simulink model "NGGenset_Test_System"  (Simulink 8.1)
settings: Solver=ode3  SolverMode=SingleTasking  StartTime=0.0  StopTime=150  FixedStep=Ts  RelTol=1e-3
PostLoadFcn:
  | Ts=50e-6;
InitFcn:
  | Ts=50e-6;
undefined symbols (not defined in the file): another_event_name, DiscIntNeverNeededParam, fdesignblkfcn, gcbh, Gen_900kW_external_control, HIL_GenSet, Left, my_event_name, ph, type, V
libraries: powerlib x47, simulink x40, powerlib_extras x28, rtio_opalrt_common x21, dspsigops x7, breakers_1ph_3ph x7, rtio_generic_modbus x7, simulink_extras x6, cables_lib x5, rteventslib x4, rtlab x3, discretizing x2
(part 3 of 5)

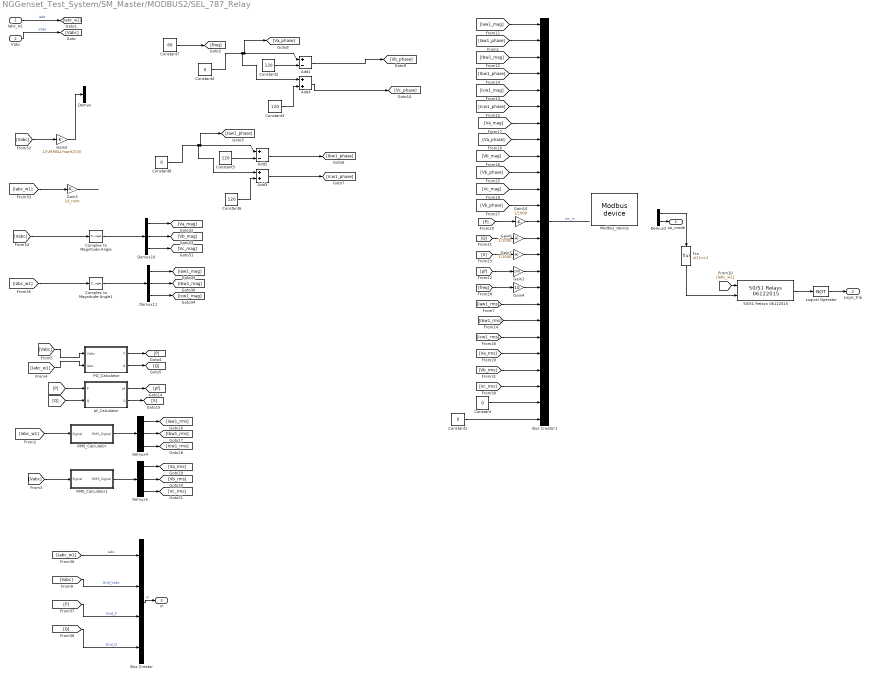
== system NGGenset_Test_System/SM_Master/MODBUS2/SEL_787_Relay ==
  Iabc_w1 : Inport
  Vabc : Inport  Port=2
  50/51 Relays 06122015 : breakers_1ph_3ph/50//51 Relays 06122015  TOC=TOC  IOC=IOC  Ts=Ts
  Add1 : Sum  Inputs=+-
  Add2 : Sum  Inputs=+-
  Add3 : Sum
  Add4 : Sum
  Bus Creator : BusCreator
  Bus Creator1 : BusCreator  Inputs=25
  Complex to Magnitude-Angle : ComplexToMagnitudeAngle  Output=Magnitude
  Complex to Magnitude-Angle1 : ComplexToMagnitudeAngle  Output=Magnitude
  Constant{,1,4,8} (4 alike) : Constant  Value=0
  Constant{2..3,5..6} (4 alike) : Constant  Value=120
  Constant7 : Constant  Value=60
  Demux{,4..5,10..11} (5 alike) : Demux  Outputs=3
  Demux2 : Demux  Outputs=2
  Fcn : Fcn  Expr=u(1)==1
  Gain1 : Gain  Gain=100
  Gain10 : Gain  Gain=1/1000
  Gain2 : Gain  Gain=1/(VRMSLL*sqrt(2/3))
  Gain3 : Gain  Gain=1/I_nom
  Gain4 : Gain  Gain=10
  Gain6 : Gain  Gain=1/1000
  Gain7 : Gain  Gain=1/1000
  Logical Operator : Logic  Operator=NOT  AllPortsSameDT=off  OutDataTypeStr=boolean
  Modbus_device : rtio_generic_modbus/Modbus device  conf_name=relay_slave_cfg2.opal  conf_name_mask=relay_slave_cfg2.xls  sample_time=Ts
  PQ_Calculator : Subsystem
  RMS_Calculator : Subsystem
  RMS_Calculator1 : Subsystem
  pf_Calculator : Subsystem
  op_mode : Outport
  Logic_trip : Outport  Port=2
  m : Outport  Port=3
  wires:
  Gain4/1 -> Bus Creator1/17
  Gain1/1 -> Bus Creator1/16
  [pf] -> Gain1/1
  [freq] -> Gain4/1
  Constant4/1 -> Add4/1, [Va_phase], Add1/1
  Add4/1 -> [Vc_phase]
  Add1/1 -> [Vb_phase]
  Constant3/1 -> Add4/2
  Constant2/1 -> Add1/2
  Constant8/1 -> Add3/1, [Iaw1_phase], Add2/1
  Add3/1 -> [Icw1_phase]
  Add2/1 -> [Ibw1_phase]
  Constant6/1 -> Add3/2
  Constant5/1 -> Add2/2
  Constant7/1 -> [freq]
  pf_Calculator/2(S) -> [S]
  Bus Creator1/1 -> ?  "sm_in"
  ? -> Demux2/1
  [Q] -> Bus Creator/4  "Grid_Q"
  [P] -> Bus Creator/3  "Grid_P"
  [Vabc] -> Bus Creator/2  "Grid_Vabc"
  [Iabc_w1] -> Bus Creator/1  "Iabc"
  Bus Creator/1 -> m/1  "m"
  Iabc_w1/1 -> [Iabc_w1]  "Iabc"
  Vabc/1 -> [Vabc]  "Vabc"
  [Vabc] -> PQ_Calculator/1(Vabc)
  [Iabc_w1] -> PQ_Calculator/2(Iabc)
  [Iaw1_mag] -> Bus Creator1/1
  [P] -> Gain10/1
  [Q] -> Gain6/1
  [S] -> Gain7/1
  pf_Calculator/1(pf) -> [pf]
  [P] -> pf_Calculator/1(P)
  [Q] -> pf_Calculator/2(Q)
  PQ_Calculator/1(P) -> [P]
  PQ_Calculator/2(Q) -> [Q]
  [Iabc_w1] -> RMS_Calculator/1(Signal)
  [Vabc] -> RMS_Calculator1/1(Signal)
  RMS_Calculator/1(RMS_Signal) -> Demux4/1
  RMS_Calculator1/1(RMS_Signal) -> Demux5/1
  Demux4/3 -> [Icw1_rms]
  Demux4/2 -> [Ibw1_rms]
  Demux4/1 -> [Iaw1_rms]
  Demux5/1 -> [Va_rms]
  Demux5/2 -> [Vb_rms]
  Demux5/3 -> [Vc_rms]
  Demux2/1 -> Fcn/1
  Fcn/1 -> 50/51 Relays 06122015/2
  [Iabc_w1] -> 50/51 Relays 06122015/1
  50/51 Relays 06122015/1 -> Logical Operator/1
  [Ibw1_mag] -> Bus Creator1/3
  [Icw1_mag] -> Bus Creator1/5
  [Va_mag] -> Bus Creator1/7
  [Vb_mag] -> Bus Creator1/9
  [Vc_mag] -> Bus Creator1/11
  Gain10/1 -> Bus Creator1/13
  Gain6/1 -> Bus Creator1/14
  Gain7/1 -> Bus Creator1/15
  [Iaw1_rms] -> Bus Creator1/18
  [Icw1_rms] -> Bus Creator1/20
  [Ibw1_rms] -> Bus Creator1/19
  [Va_rms] -> Bus Creator1/21
  [Vb_rms] -> Bus Creator1/22
  [Vc_rms] -> Bus Creator1/23
  Logical Operator/1 -> Logic_trip/1
  Demux2/2 -> op_mode/1
  [Iaw1_phase] -> Bus Creator1/2
  [Ibw1_phase] -> Bus Creator1/4
  [Icw1_phase] -> Bus Creator1/6
  [Va_phase] -> Bus Creator1/8
  [Vb_phase] -> Bus Creator1/10
  [Vb_phase] -> Bus Creator1/12
  Constant/1 -> Bus Creator1/24
  Constant1/1 -> Bus Creator1/25
  [Vabc] -> Gain2/1
  Gain2/1 -> Demux/1
  [Iabc_w1] -> Gain3/1
  Gain3/1 -> ?
  Demux10/1 -> [Va_mag]
  Demux10/2 -> [Vb_mag]
  Demux10/3 -> [Vc_mag]
  Complex to Magnitude-Angle/1 -> Demux10/1
  [Vabc] -> Complex to Magnitude-Angle/1
  Complex to Magnitude-Angle1/1 -> Demux11/1
  [Iabc_w1] -> Complex to Magnitude-Angle1/1
  Demux11/1 -> [Iaw1_mag]
  Demux11/2 -> [Ibw1_mag]
  Demux11/3 -> [Icw1_mag]

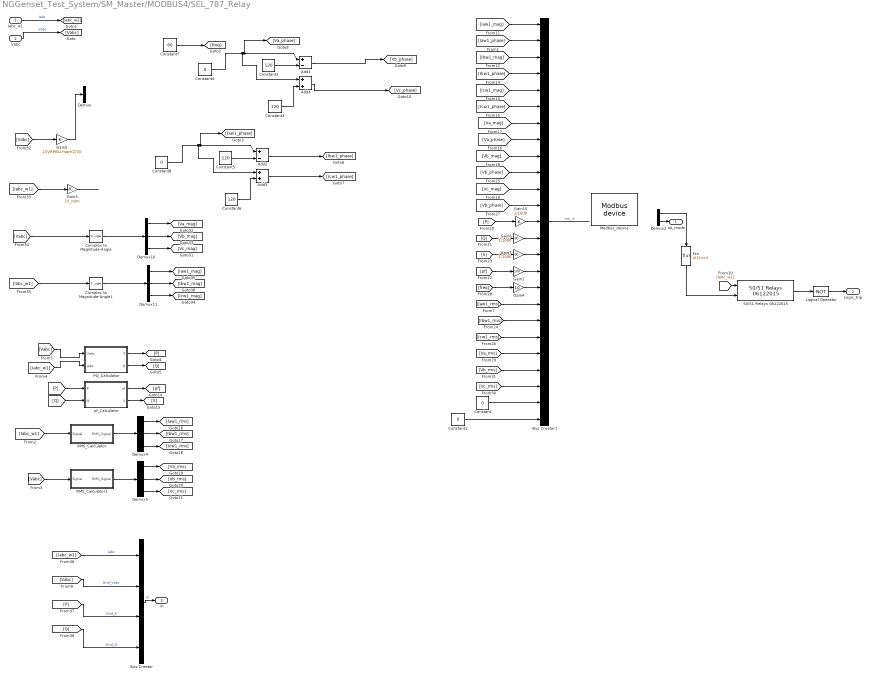
== system NGGenset_Test_System/SM_Master/MODBUS4/SEL_787_Relay ==
  Iabc_w1 : Inport
  Vabc : Inport  Port=2
  50/51 Relays 06122015 : breakers_1ph_3ph/50//51 Relays 06122015  TOC=TOC  IOC=IOC  Ts=Ts
  Add1 : Sum  Inputs=+-
  Add2 : Sum  Inputs=+-
  Add3 : Sum
  Add4 : Sum
  Bus Creator : BusCreator
  Bus Creator1 : BusCreator  Inputs=25
  Complex to Magnitude-Angle : ComplexToMagnitudeAngle  Output=Magnitude
  Complex to Magnitude-Angle1 : ComplexToMagnitudeAngle  Output=Magnitude
  Constant{,1,4,8} (4 alike) : Constant  Value=0
  Constant{2..3,5..6} (4 alike) : Constant  Value=120
  Constant7 : Constant  Value=60
  Demux{,4..5,10..11} (5 alike) : Demux  Outputs=3
  Demux2 : Demux  Outputs=2
  Fcn : Fcn  Expr=u(1)==1
  Gain1 : Gain  Gain=100
  Gain10 : Gain  Gain=1/1000
  Gain2 : Gain  Gain=1/(VRMSLL*sqrt(2/3))
  Gain3 : Gain  Gain=1/I_nom
  Gain4 : Gain  Gain=10
  Gain6 : Gain  Gain=1/1000
  Gain7 : Gain  Gain=1/1000
  Logical Operator : Logic  Operator=NOT  AllPortsSameDT=off  OutDataTypeStr=boolean
  Modbus_device : rtio_generic_modbus/Modbus device  conf_name=relay_slave_cfg4.opal  conf_name_mask=relay_slave_cfg4.xls  sample_time=Ts
  PQ_Calculator : Subsystem
  RMS_Calculator : Subsystem
  RMS_Calculator1 : Subsystem
  pf_Calculator : Subsystem
  op_mode : Outport
  Logic_trip : Outport  Port=2
  m : Outport  Port=3
  wires:
  Gain4/1 -> Bus Creator1/17
  Gain1/1 -> Bus Creator1/16
  [pf] -> Gain1/1
  [freq] -> Gain4/1
  Constant4/1 -> Add4/1, [Va_phase], Add1/1
  Add4/1 -> [Vc_phase]
  Add1/1 -> [Vb_phase]
  Constant3/1 -> Add4/2
  Constant2/1 -> Add1/2
  Constant8/1 -> Add3/1, [Iaw1_phase], Add2/1
  Add3/1 -> [Icw1_phase]
  Add2/1 -> [Ibw1_phase]
  Constant6/1 -> Add3/2
  Constant5/1 -> Add2/2
  Constant7/1 -> [freq]
  pf_Calculator/2(S) -> [S]
  Bus Creator1/1 -> ?  "sm_in"
  ? -> Demux2/1
  [Q] -> Bus Creator/4  "Grid_Q"
  [P] -> Bus Creator/3  "Grid_P"
  [Vabc] -> Bus Creator/2  "Grid_Vabc"
  [Iabc_w1] -> Bus Creator/1  "Iabc"
  Bus Creator/1 -> m/1  "m"
  Iabc_w1/1 -> [Iabc_w1]  "Iabc"
  Vabc/1 -> [Vabc]  "Vabc"
  [Vabc] -> PQ_Calculator/1(Vabc)
  [Iabc_w1] -> PQ_Calculator/2(Iabc)
  [Iaw1_mag] -> Bus Creator1/1
  [P] -> Gain10/1
  [Q] -> Gain6/1
  [S] -> Gain7/1
  pf_Calculator/1(pf) -> [pf]
  [P] -> pf_Calculator/1(P)
  [Q] -> pf_Calculator/2(Q)
  PQ_Calculator/1(P) -> [P]
  PQ_Calculator/2(Q) -> [Q]
  [Iabc_w1] -> RMS_Calculator/1(Signal)
  [Vabc] -> RMS_Calculator1/1(Signal)
  RMS_Calculator/1(RMS_Signal) -> Demux4/1
  RMS_Calculator1/1(RMS_Signal) -> Demux5/1
  Demux4/3 -> [Icw1_rms]
  Demux4/2 -> [Ibw1_rms]
  Demux4/1 -> [Iaw1_rms]
  Demux5/1 -> [Va_rms]
  Demux5/2 -> [Vb_rms]
  Demux5/3 -> [Vc_rms]
  Demux2/1 -> Fcn/1
  Fcn/1 -> 50/51 Relays 06122015/2
  [Iabc_w1] -> 50/51 Relays 06122015/1
  50/51 Relays 06122015/1 -> Logical Operator/1
  [Ibw1_mag] -> Bus Creator1/3
  [Icw1_mag] -> Bus Creator1/5
  [Va_mag] -> Bus Creator1/7
  [Vb_mag] -> Bus Creator1/9
  [Vc_mag] -> Bus Creator1/11
  Gain10/1 -> Bus Creator1/13
  Gain6/1 -> Bus Creator1/14
  Gain7/1 -> Bus Creator1/15
  [Iaw1_rms] -> Bus Creator1/18
  [Icw1_rms] -> Bus Creator1/20
  [Ibw1_rms] -> Bus Creator1/19
  [Va_rms] -> Bus Creator1/21
  [Vb_rms] -> Bus Creator1/22
  [Vc_rms] -> Bus Creator1/23
  Logical Operator/1 -> Logic_trip/1
  Demux2/2 -> op_mode/1
  [Iaw1_phase] -> Bus Creator1/2
  [Ibw1_phase] -> Bus Creator1/4
  [Icw1_phase] -> Bus Creator1/6
  [Va_phase] -> Bus Creator1/8
  [Vb_phase] -> Bus Creator1/10
  [Vb_phase] -> Bus Creator1/12
  Constant/1 -> Bus Creator1/24
  Constant1/1 -> Bus Creator1/25
  [Vabc] -> Gain2/1
  Gain2/1 -> Demux/1
  [Iabc_w1] -> Gain3/1
  Gain3/1 -> ?
  Demux10/1 -> [Va_mag]
  Demux10/2 -> [Vb_mag]
  Demux10/3 -> [Vc_mag]
  Complex to Magnitude-Angle/1 -> Demux10/1
  [Vabc] -> Complex to Magnitude-Angle/1
  Complex to Magnitude-Angle1/1 -> Demux11/1
  [Iabc_w1] -> Complex to Magnitude-Angle1/1
  Demux11/1 -> [Iaw1_mag]
  Demux11/2 -> [Ibw1_mag]
  Demux11/3 -> [Icw1_mag]

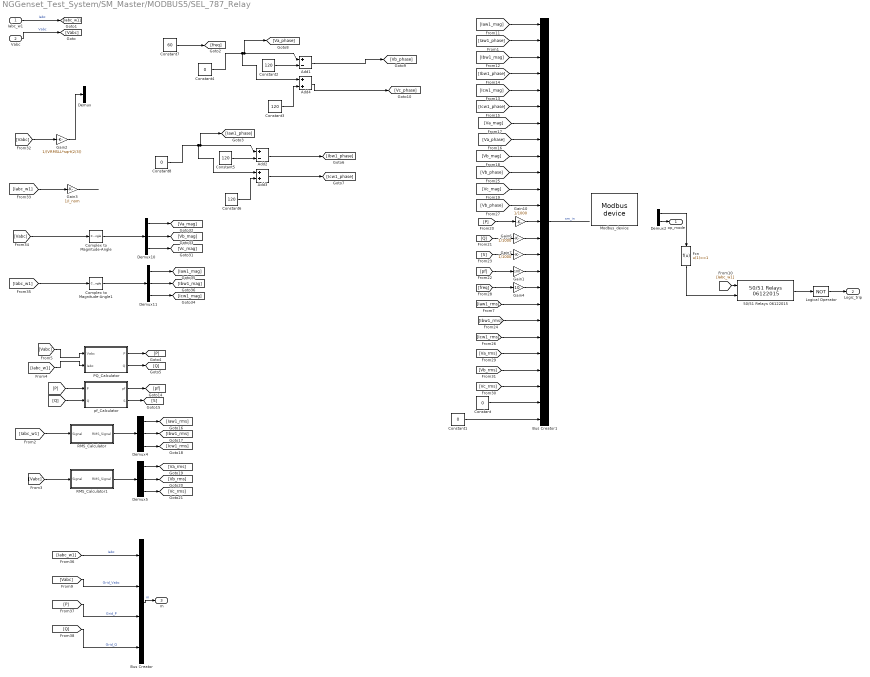
== system NGGenset_Test_System/SM_Master/MODBUS5/SEL_787_Relay ==
  Iabc_w1 : Inport
  Vabc : Inport  Port=2
  50/51 Relays 06122015 : breakers_1ph_3ph/50//51 Relays 06122015  TOC=TOC  IOC=IOC  Ts=Ts
  Add1 : Sum  Inputs=+-
  Add2 : Sum  Inputs=+-
  Add3 : Sum
  Add4 : Sum
  Bus Creator : BusCreator
  Bus Creator1 : BusCreator  Inputs=25
  Complex to Magnitude-Angle : ComplexToMagnitudeAngle  Output=Magnitude
  Complex to Magnitude-Angle1 : ComplexToMagnitudeAngle  Output=Magnitude
  Constant{,1,4,8} (4 alike) : Constant  Value=0
  Constant{2..3,5..6} (4 alike) : Constant  Value=120
  Constant7 : Constant  Value=60
  Demux{,4..5,10..11} (5 alike) : Demux  Outputs=3
  Demux2 : Demux  Outputs=2
  Fcn : Fcn  Expr=u(1)==1
  Gain1 : Gain  Gain=100
  Gain10 : Gain  Gain=1/1000
  Gain2 : Gain  Gain=1/(VRMSLL*sqrt(2/3))
  Gain3 : Gain  Gain=1/I_nom
  Gain4 : Gain  Gain=10
  Gain6 : Gain  Gain=1/1000
  Gain7 : Gain  Gain=1/1000
  Logical Operator : Logic  Operator=NOT  AllPortsSameDT=off  OutDataTypeStr=boolean
  Modbus_device : rtio_generic_modbus/Modbus device  conf_name=relay_slave_cfg5.opal  conf_name_mask=relay_slave_cfg5.xls  sample_time=Ts
  PQ_Calculator : Subsystem
  RMS_Calculator : Subsystem
  RMS_Calculator1 : Subsystem
  pf_Calculator : Subsystem
  op_mode : Outport
  Logic_trip : Outport  Port=2
  m : Outport  Port=3
  wires:
  Gain4/1 -> Bus Creator1/17
  Gain1/1 -> Bus Creator1/16
  [pf] -> Gain1/1
  [freq] -> Gain4/1
  Constant4/1 -> Add4/1, [Va_phase], Add1/1
  Add4/1 -> [Vc_phase]
  Add1/1 -> [Vb_phase]
  Constant3/1 -> Add4/2
  Constant2/1 -> Add1/2
  Constant8/1 -> Add3/1, [Iaw1_phase], Add2/1
  Add3/1 -> [Icw1_phase]
  Add2/1 -> [Ibw1_phase]
  Constant6/1 -> Add3/2
  Constant5/1 -> Add2/2
  Constant7/1 -> [freq]
  pf_Calculator/2(S) -> [S]
  Bus Creator1/1 -> ?  "sm_in"
  ? -> Demux2/1
  [Q] -> Bus Creator/4  "Grid_Q"
  [P] -> Bus Creator/3  "Grid_P"
  [Vabc] -> Bus Creator/2  "Grid_Vabc"
  [Iabc_w1] -> Bus Creator/1  "Iabc"
  Bus Creator/1 -> m/1  "m"
  Iabc_w1/1 -> [Iabc_w1]  "Iabc"
  Vabc/1 -> [Vabc]  "Vabc"
  [Vabc] -> PQ_Calculator/1(Vabc)
  [Iabc_w1] -> PQ_Calculator/2(Iabc)
  [Iaw1_mag] -> Bus Creator1/1
  [P] -> Gain10/1
  [Q] -> Gain6/1
  [S] -> Gain7/1
  pf_Calculator/1(pf) -> [pf]
  [P] -> pf_Calculator/1(P)
  [Q] -> pf_Calculator/2(Q)
  PQ_Calculator/1(P) -> [P]
  PQ_Calculator/2(Q) -> [Q]
  [Iabc_w1] -> RMS_Calculator/1(Signal)
  [Vabc] -> RMS_Calculator1/1(Signal)
  RMS_Calculator/1(RMS_Signal) -> Demux4/1
  RMS_Calculator1/1(RMS_Signal) -> Demux5/1
  Demux4/3 -> [Icw1_rms]
  Demux4/2 -> [Ibw1_rms]
  Demux4/1 -> [Iaw1_rms]
  Demux5/1 -> [Va_rms]
  Demux5/2 -> [Vb_rms]
  Demux5/3 -> [Vc_rms]
  Demux2/1 -> Fcn/1
  Fcn/1 -> 50/51 Relays 06122015/2
  [Iabc_w1] -> 50/51 Relays 06122015/1
  50/51 Relays 06122015/1 -> Logical Operator/1
  [Ibw1_mag] -> Bus Creator1/3
  [Icw1_mag] -> Bus Creator1/5
  [Va_mag] -> Bus Creator1/7
  [Vb_mag] -> Bus Creator1/9
  [Vc_mag] -> Bus Creator1/11
  Gain10/1 -> Bus Creator1/13
  Gain6/1 -> Bus Creator1/14
  Gain7/1 -> Bus Creator1/15
  [Iaw1_rms] -> Bus Creator1/18
  [Icw1_rms] -> Bus Creator1/20
  [Ibw1_rms] -> Bus Creator1/19
  [Va_rms] -> Bus Creator1/21
  [Vb_rms] -> Bus Creator1/22
  [Vc_rms] -> Bus Creator1/23
  Logical Operator/1 -> Logic_trip/1
  Demux2/2 -> op_mode/1
  [Iaw1_phase] -> Bus Creator1/2
  [Ibw1_phase] -> Bus Creator1/4
  [Icw1_phase] -> Bus Creator1/6
  [Va_phase] -> Bus Creator1/8
  [Vb_phase] -> Bus Creator1/10
  [Vb_phase] -> Bus Creator1/12
  Constant/1 -> Bus Creator1/24
  Constant1/1 -> Bus Creator1/25
  [Vabc] -> Gain2/1
  Gain2/1 -> Demux/1
  [Iabc_w1] -> Gain3/1
  Gain3/1 -> ?
  Demux10/1 -> [Va_mag]
  Demux10/2 -> [Vb_mag]
  Demux10/3 -> [Vc_mag]
  Complex to Magnitude-Angle/1 -> Demux10/1
  [Vabc] -> Complex to Magnitude-Angle/1
  Complex to Magnitude-Angle1/1 -> Demux11/1
  [Iabc_w1] -> Complex to Magnitude-Angle1/1
  Demux11/1 -> [Iaw1_mag]
  Demux11/2 -> [Ibw1_mag]
  Demux11/3 -> [Icw1_mag]

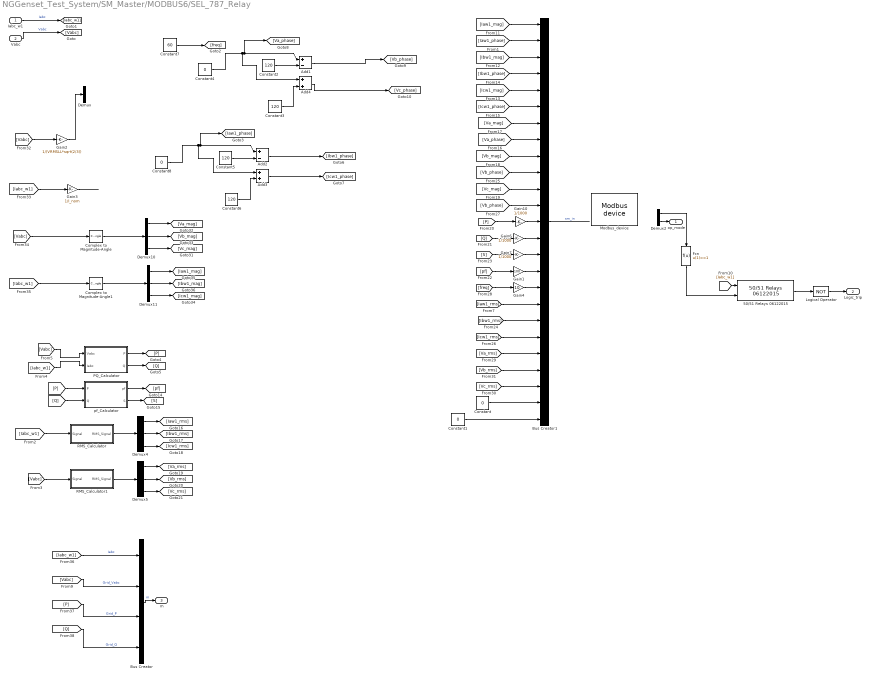
== system NGGenset_Test_System/SM_Master/MODBUS6/SEL_787_Relay ==
  Iabc_w1 : Inport
  Vabc : Inport  Port=2
  50/51 Relays 06122015 : breakers_1ph_3ph/50//51 Relays 06122015  TOC=TOC  IOC=IOC  Ts=Ts
  Add1 : Sum  Inputs=+-
  Add2 : Sum  Inputs=+-
  Add3 : Sum
  Add4 : Sum
  Bus Creator : BusCreator
  Bus Creator1 : BusCreator  Inputs=25
  Complex to Magnitude-Angle : ComplexToMagnitudeAngle  Output=Magnitude
  Complex to Magnitude-Angle1 : ComplexToMagnitudeAngle  Output=Magnitude
  Constant{,1,4,8} (4 alike) : Constant  Value=0
  Constant{2..3,5..6} (4 alike) : Constant  Value=120
  Constant7 : Constant  Value=60
  Demux{,4..5,10..11} (5 alike) : Demux  Outputs=3
  Demux2 : Demux  Outputs=2
  Fcn : Fcn  Expr=u(1)==1
  Gain1 : Gain  Gain=100
  Gain10 : Gain  Gain=1/1000
  Gain2 : Gain  Gain=1/(VRMSLL*sqrt(2/3))
  Gain3 : Gain  Gain=1/I_nom
  Gain4 : Gain  Gain=10
  Gain6 : Gain  Gain=1/1000
  Gain7 : Gain  Gain=1/1000
  Logical Operator : Logic  Operator=NOT  AllPortsSameDT=off  OutDataTypeStr=boolean
  Modbus_device : rtio_generic_modbus/Modbus device  conf_name=relay_slave_cfg5.opal  conf_name_mask=relay_slave_cfg5.xls  sample_time=Ts
  PQ_Calculator : Subsystem
  RMS_Calculator : Subsystem
  RMS_Calculator1 : Subsystem
  pf_Calculator : Subsystem
  op_mode : Outport
  Logic_trip : Outport  Port=2
  m : Outport  Port=3
  wires:
  Gain4/1 -> Bus Creator1/17
  Gain1/1 -> Bus Creator1/16
  [pf] -> Gain1/1
  [freq] -> Gain4/1
  Constant4/1 -> Add4/1, [Va_phase], Add1/1
  Add4/1 -> [Vc_phase]
  Add1/1 -> [Vb_phase]
  Constant3/1 -> Add4/2
  Constant2/1 -> Add1/2
  Constant8/1 -> Add3/1, [Iaw1_phase], Add2/1
  Add3/1 -> [Icw1_phase]
  Add2/1 -> [Ibw1_phase]
  Constant6/1 -> Add3/2
  Constant5/1 -> Add2/2
  Constant7/1 -> [freq]
  pf_Calculator/2(S) -> [S]
  Bus Creator1/1 -> ?  "sm_in"
  ? -> Demux2/1
  [Q] -> Bus Creator/4  "Grid_Q"
  [P] -> Bus Creator/3  "Grid_P"
  [Vabc] -> Bus Creator/2  "Grid_Vabc"
  [Iabc_w1] -> Bus Creator/1  "Iabc"
  Bus Creator/1 -> m/1  "m"
  Iabc_w1/1 -> [Iabc_w1]  "Iabc"
  Vabc/1 -> [Vabc]  "Vabc"
  [Vabc] -> PQ_Calculator/1(Vabc)
  [Iabc_w1] -> PQ_Calculator/2(Iabc)
  [Iaw1_mag] -> Bus Creator1/1
  [P] -> Gain10/1
  [Q] -> Gain6/1
  [S] -> Gain7/1
  pf_Calculator/1(pf) -> [pf]
  [P] -> pf_Calculator/1(P)
  [Q] -> pf_Calculator/2(Q)
  PQ_Calculator/1(P) -> [P]
  PQ_Calculator/2(Q) -> [Q]
  [Iabc_w1] -> RMS_Calculator/1(Signal)
  [Vabc] -> RMS_Calculator1/1(Signal)
  RMS_Calculator/1(RMS_Signal) -> Demux4/1
  RMS_Calculator1/1(RMS_Signal) -> Demux5/1
  Demux4/3 -> [Icw1_rms]
  Demux4/2 -> [Ibw1_rms]
  Demux4/1 -> [Iaw1_rms]
  Demux5/1 -> [Va_rms]
  Demux5/2 -> [Vb_rms]
  Demux5/3 -> [Vc_rms]
  Demux2/1 -> Fcn/1
  Fcn/1 -> 50/51 Relays 06122015/2
  [Iabc_w1] -> 50/51 Relays 06122015/1
  50/51 Relays 06122015/1 -> Logical Operator/1
  [Ibw1_mag] -> Bus Creator1/3
  [Icw1_mag] -> Bus Creator1/5
  [Va_mag] -> Bus Creator1/7
  [Vb_mag] -> Bus Creator1/9
  [Vc_mag] -> Bus Creator1/11
  Gain10/1 -> Bus Creator1/13
  Gain6/1 -> Bus Creator1/14
  Gain7/1 -> Bus Creator1/15
  [Iaw1_rms] -> Bus Creator1/18
  [Icw1_rms] -> Bus Creator1/20
  [Ibw1_rms] -> Bus Creator1/19
  [Va_rms] -> Bus Creator1/21
  [Vb_rms] -> Bus Creator1/22
  [Vc_rms] -> Bus Creator1/23
  Logical Operator/1 -> Logic_trip/1
  Demux2/2 -> op_mode/1
  [Iaw1_phase] -> Bus Creator1/2
  [Ibw1_phase] -> Bus Creator1/4
  [Icw1_phase] -> Bus Creator1/6
  [Va_phase] -> Bus Creator1/8
  [Vb_phase] -> Bus Creator1/10
  [Vb_phase] -> Bus Creator1/12
  Constant/1 -> Bus Creator1/24
  Constant1/1 -> Bus Creator1/25
  [Vabc] -> Gain2/1
  Gain2/1 -> Demux/1
  [Iabc_w1] -> Gain3/1
  Gain3/1 -> ?
  Demux10/1 -> [Va_mag]
  Demux10/2 -> [Vb_mag]
  Demux10/3 -> [Vc_mag]
  Complex to Magnitude-Angle/1 -> Demux10/1
  [Vabc] -> Complex to Magnitude-Angle/1
  Complex to Magnitude-Angle1/1 -> Demux11/1
  [Iabc_w1] -> Complex to Magnitude-Angle1/1
  Demux11/1 -> [Iaw1_mag]
  Demux11/2 -> [Ibw1_mag]
  Demux11/3 -> [Icw1_mag]

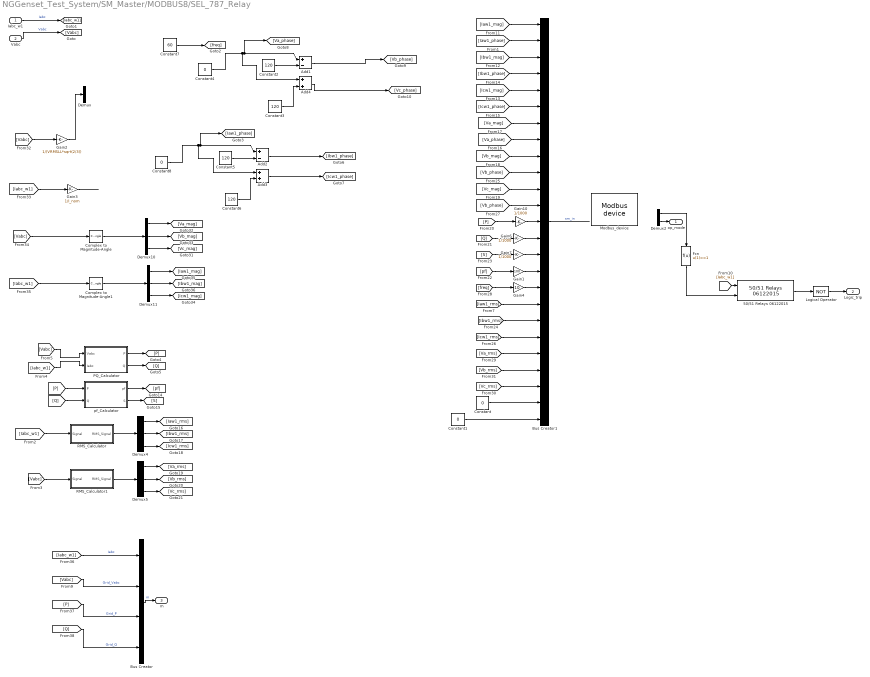
== system NGGenset_Test_System/SM_Master/MODBUS8/SEL_787_Relay ==
  Iabc_w1 : Inport
  Vabc : Inport  Port=2
  50/51 Relays 06122015 : breakers_1ph_3ph/50//51 Relays 06122015  TOC=TOC  IOC=IOC  Ts=Ts
  Add1 : Sum  Inputs=+-
  Add2 : Sum  Inputs=+-
  Add3 : Sum
  Add4 : Sum
  Bus Creator : BusCreator
  Bus Creator1 : BusCreator  Inputs=25
  Complex to Magnitude-Angle : ComplexToMagnitudeAngle  Output=Magnitude
  Complex to Magnitude-Angle1 : ComplexToMagnitudeAngle  Output=Magnitude
  Constant{,1,4,8} (4 alike) : Constant  Value=0
  Constant{2..3,5..6} (4 alike) : Constant  Value=120
  Constant7 : Constant  Value=60
  Demux{,4..5,10..11} (5 alike) : Demux  Outputs=3
  Demux2 : Demux  Outputs=2
  Fcn : Fcn  Expr=u(1)==1
  Gain1 : Gain  Gain=100
  Gain10 : Gain  Gain=1/1000
  Gain2 : Gain  Gain=1/(VRMSLL*sqrt(2/3))
  Gain3 : Gain  Gain=1/I_nom
  Gain4 : Gain  Gain=10
  Gain6 : Gain  Gain=1/1000
  Gain7 : Gain  Gain=1/1000
  Logical Operator : Logic  Operator=NOT  AllPortsSameDT=off  OutDataTypeStr=boolean
  Modbus_device : rtio_generic_modbus/Modbus device  conf_name=relay_slave_cfg8.opal  conf_name_mask=relay_slave_cfg8.xls  sample_time=Ts
  PQ_Calculator : Subsystem
  RMS_Calculator : Subsystem
  RMS_Calculator1 : Subsystem
  pf_Calculator : Subsystem
  op_mode : Outport
  Logic_trip : Outport  Port=2
  m : Outport  Port=3
  wires:
  Gain4/1 -> Bus Creator1/17
  Gain1/1 -> Bus Creator1/16
  [pf] -> Gain1/1
  [freq] -> Gain4/1
  Constant4/1 -> Add4/1, [Va_phase], Add1/1
  Add4/1 -> [Vc_phase]
  Add1/1 -> [Vb_phase]
  Constant3/1 -> Add4/2
  Constant2/1 -> Add1/2
  Constant8/1 -> Add3/1, [Iaw1_phase], Add2/1
  Add3/1 -> [Icw1_phase]
  Add2/1 -> [Ibw1_phase]
  Constant6/1 -> Add3/2
  Constant5/1 -> Add2/2
  Constant7/1 -> [freq]
  pf_Calculator/2(S) -> [S]
  Bus Creator1/1 -> ?  "sm_in"
  ? -> Demux2/1
  [Q] -> Bus Creator/4  "Grid_Q"
  [P] -> Bus Creator/3  "Grid_P"
  [Vabc] -> Bus Creator/2  "Grid_Vabc"
  [Iabc_w1] -> Bus Creator/1  "Iabc"
  Bus Creator/1 -> m/1  "m"
  Iabc_w1/1 -> [Iabc_w1]  "Iabc"
  Vabc/1 -> [Vabc]  "Vabc"
  [Vabc] -> PQ_Calculator/1(Vabc)
  [Iabc_w1] -> PQ_Calculator/2(Iabc)
  [Iaw1_mag] -> Bus Creator1/1
  [P] -> Gain10/1
  [Q] -> Gain6/1
  [S] -> Gain7/1
  pf_Calculator/1(pf) -> [pf]
  [P] -> pf_Calculator/1(P)
  [Q] -> pf_Calculator/2(Q)
  PQ_Calculator/1(P) -> [P]
  PQ_Calculator/2(Q) -> [Q]
  [Iabc_w1] -> RMS_Calculator/1(Signal)
  [Vabc] -> RMS_Calculator1/1(Signal)
  RMS_Calculator/1(RMS_Signal) -> Demux4/1
  RMS_Calculator1/1(RMS_Signal) -> Demux5/1
  Demux4/3 -> [Icw1_rms]
  Demux4/2 -> [Ibw1_rms]
  Demux4/1 -> [Iaw1_rms]
  Demux5/1 -> [Va_rms]
  Demux5/2 -> [Vb_rms]
  Demux5/3 -> [Vc_rms]
  Demux2/1 -> Fcn/1
  Fcn/1 -> 50/51 Relays 06122015/2
  [Iabc_w1] -> 50/51 Relays 06122015/1
  50/51 Relays 06122015/1 -> Logical Operator/1
  [Ibw1_mag] -> Bus Creator1/3
  [Icw1_mag] -> Bus Creator1/5
  [Va_mag] -> Bus Creator1/7
  [Vb_mag] -> Bus Creator1/9
  [Vc_mag] -> Bus Creator1/11
  Gain10/1 -> Bus Creator1/13
  Gain6/1 -> Bus Creator1/14
  Gain7/1 -> Bus Creator1/15
  [Iaw1_rms] -> Bus Creator1/18
  [Icw1_rms] -> Bus Creator1/20
  [Ibw1_rms] -> Bus Creator1/19
  [Va_rms] -> Bus Creator1/21
  [Vb_rms] -> Bus Creator1/22
  [Vc_rms] -> Bus Creator1/23
  Logical Operator/1 -> Logic_trip/1
  Demux2/2 -> op_mode/1
  [Iaw1_phase] -> Bus Creator1/2
  [Ibw1_phase] -> Bus Creator1/4
  [Icw1_phase] -> Bus Creator1/6
  [Va_phase] -> Bus Creator1/8
  [Vb_phase] -> Bus Creator1/10
  [Vb_phase] -> Bus Creator1/12
  Constant/1 -> Bus Creator1/24
  Constant1/1 -> Bus Creator1/25
  [Vabc] -> Gain2/1
  Gain2/1 -> Demux/1
  [Iabc_w1] -> Gain3/1
  Gain3/1 -> ?
  Demux10/1 -> [Va_mag]
  Demux10/2 -> [Vb_mag]
  Demux10/3 -> [Vc_mag]
  Complex to Magnitude-Angle/1 -> Demux10/1
  [Vabc] -> Complex to Magnitude-Angle/1
  Complex to Magnitude-Angle1/1 -> Demux11/1
  [Iabc_w1] -> Complex to Magnitude-Angle1/1
  Demux11/1 -> [Iaw1_mag]
  Demux11/2 -> [Ibw1_mag]
  Demux11/3 -> [Icw1_mag]

== system NGGenset_Test_System/SC_Console/Woodward/16TSDIn/16 TSDOut GR3/Din/Dout ch16-23 ==
  Bus Creator3 : BusCreator  Inputs=8
  times17 : Constant  Value=[0.05 0.15 0.25 0.35]
  times18 : Constant  Value=[0.1 0.2 0.3 0.4]
  times19 : Constant  Value=[0.15 0.25 0.35 0.45]
  times20 : Constant  Value=[0.2 0.3 0.4 0.5]
  times21 : Constant  Value=[0.25 0.35 0.45 0.55]
  times22 : Constant  Value=[0.3 0.4 0.5 0.6]
  times23 : Constant  Value=[0.3 0.4 0.5 0.6]
  times24 : Constant  Value=[0 0.1 0.2 0.3]
  Out1 : Outport
  wires:
  Bus Creator3/1 -> Out1/1
  times23/1 -> Bus Creator3/8  "times24"
  times22/1 -> Bus Creator3/7  "times23"
  times21/1 -> Bus Creator3/6  "times22"
  times20/1 -> Bus Creator3/5  "times21"
  times19/1 -> Bus Creator3/4  "times20"
  times18/1 -> Bus Creator3/3  "times19"
  times17/1 -> Bus Creator3/2  "times18"
  times24/1 -> Bus Creator3/1  "times17"

== system NGGenset_Test_System/SC_Console/Woodward/16TSDIn/16 TSDOut GR3/Din/Dout ch24-31 ==
  Bus Creator4 : BusCreator  Inputs=8
  times25 : Constant  Value=[0.05 0.15 0.25 0.35]
  times26 : Constant  Value=[0.1 0.2 0.3 0.4]
  times27 : Constant  Value=[0.15 0.25 0.35 0.45]
  times28 : Constant  Value=[0.2 0.3 0.4 0.5]
  times29 : Constant  Value=[0.25 0.35 0.45 0.55]
  times30 : Constant  Value=[0.3 0.4 0.5 0.6]
  times31 : Constant  Value=[0.3 0.4 0.5 0.6]
  times32 : Constant  Value=[0 0.1 0.2 0.3]
  Out1 : Outport
  wires:
  Bus Creator4/1 -> Out1/1
  times31/1 -> Bus Creator4/8  "times32"
  times30/1 -> Bus Creator4/7  "times31"
  times29/1 -> Bus Creator4/6  "times30"
  times28/1 -> Bus Creator4/5  "times29"
  times27/1 -> Bus Creator4/4  "times28"
  times26/1 -> Bus Creator4/3  "times27"
  times25/1 -> Bus Creator4/2  "times26"
  times32/1 -> Bus Creator4/1  "times25"

== system NGGenset_Test_System/SC_Console/Woodward/16TSDIn/16 TSDOut GR3/Dout state ctrl ==
  Bus Creator : BusCreator  Inputs=2
  Dout_CH16_CH23 : Subsystem
  Dout_CH24_CH31 : Subsystem
  Event State OUT : Outport
  wires:
  Dout_CH24_CH31/1(Dout_CH8_CH15) -> Bus Creator/2  "CH24-31"
  Dout_CH16_CH23/1(Dout_CH8_CH15) -> Bus Creator/1  "CH16-23"
  Bus Creator/1 -> Event State OUT/1

== system NGGenset_Test_System/SM_Master/Generator/GenSet_4MVA_copy1mva/4MVA Generator with  Primary Controllers ==
  wref : Inport
  Vtref : Inport  Port=2
  Enable : Inport  Port=3
  w_meas_Woodward : Inport  Port=4
  V_meas_Woodward : Inport  Port=5
  Woodward_Enable : Inport  Port=6
  Bus Creator1 : BusCreator
  Bus Creator3 : BusCreator  Inputs=3
  Bus Selector : BusSelector  OutputSignals=Vf_before,Vf_after
  Diesel Engine Speed & Voltage Control fast : Subsystem
  Synchronous Machine pu Fundamental : powerlib/Machines/Synchronous Machine pu Fundamental  PresetModel=No  MechanicalLoad=Mechanical power Pm  ShowDetailedParameters=on  RotorType=Salient-pole  NominalParameters=[4e+006 13800 60]  Stator=[0.008979 0.05 2.35 1.72]  Field=[0.00206 0.511]  Dampers2=[0.0652, 0.5134, 0.0287, 0.2553, 7.765e-3, 0.9167 ]  Dampers1=[0.2826 3.738 0.02545 0.2392]  Mechanical=[0.3468 0.009238 2]  PolePairs=2  InitialConditions="[ -99  0  0  0  0  0  0  0  0 ]"  SetSaturation=off  Saturation=[0.6404,0.7127,0.8441,0.9214,0.9956,1.082,1.19,1.316,1.457;0.7,0.7698,0.8872,0.9466,0.9969,1.046,1.1,1.151,1.201]  Units=per unit fundamental parameters  LoadFlowParameters=[1,0,0,0,0]  TsPowergui=0  TsBlock=-1  IterativeModel=Forward Euler  BusType=swing  Pref=0  Qref=0  Qmin=-inf  Qmax=inf  PLF=0  QLF=0
  A : PMIOPort  Port=1  Side=Right
  B : PMIOPort  Port=2  Side=Right
  C : PMIOPort  Port=3  Side=Right
  m : Outport
  Primary : Outport  Port=2
  wires:
  Woodward_Enable/1 -> Diesel Engine Speed & Voltage Control fast/7(Woodward Enable)
  Bus Creator3/1 -> Bus Creator1/2  "Vf"
  Bus Selector/2 -> Bus Creator3/3  "<Vf_after>"
  Bus Selector/1 -> Bus Creator3/2  "<Vf_before>"
  Diesel Engine Speed & Voltage Control fast/5(Misc) -> Bus Selector/1
  Bus Creator1/1 -> Primary/1
  Diesel Engine Speed & Voltage Control fast/4(w) -> Bus Creator1/4  "w"
  Diesel Engine Speed & Voltage Control fast/3(Vt) -> Bus Creator1/3  "vt"
  V_meas_Woodward/1 -> Diesel Engine Speed & Voltage Control fast/6(V_meas_Wood)
  w_meas_Woodward/1 -> Diesel Engine Speed & Voltage Control fast/5(w_meas_Wood)
  Synchronous Machine pu Fundamental/1 -> Diesel Engine Speed & Voltage Control fast/4(m), m/1
  Enable/1 -> Diesel Engine Speed & Voltage Control fast/3(Generator Enable)
  Diesel Engine Speed & Voltage Control fast/1(Pm) -> Bus Creator1/1, Synchronous Machine pu Fundamental/1  "Pm"
  Diesel Engine Speed & Voltage Control fast/2(Vf) -> Bus Creator3/1, Synchronous Machine pu Fundamental/2  "vf"
  wref/1 -> Diesel Engine Speed & Voltage Control fast/1(wref)
  Vtref/1 -> Diesel Engine Speed & Voltage Control fast/2(Vtref)
  connections:
  A/RConn1 -- Synchronous Machine pu Fundamental/RConn1
  B/RConn1 -- Synchronous Machine pu Fundamental/RConn2
  C/RConn1 -- Synchronous Machine pu Fundamental/RConn3

== system NGGenset_Test_System/SM_Master/Generator/GenSet_4MVA_copy1mva/Interface between Woodward Controller and simated generator ==
  note: Note: This may need a different scaling because it is the reference signal.
      | Reference has to be between 0.95 and 1.05 pu in order to be in tolerance.
  Woodward for wref : Inport
  Woodward for Vref : Inport  Port=2
  Add2 : Sum
  Add3 : Sum
  Gain2 : Gain
  Gain3 : Gain
  Mux1 : Mux  Inputs=2
  Vref_set : Constant  Value=0
  wref_set : Constant  Value=0
  wref,Vref : Outport
  wires:
  Woodward for Vref/1 -> Gain3/1
  Mux1/1 -> wref,Vref/1  "hardware"
  Woodward for wref/1 -> Gain2/1
  Add3/1 -> Mux1/2
  Vref_set/1 -> Add3/2
  Gain3/1 -> Add3/1  "bias"
  wref_set/1 -> Add2/2
  Add2/1 -> Mux1/1
  Gain2/1 -> Add2/1  "bias"

== system NGGenset_Test_System/SM_Master/Generator/GenSet_4MVA_copy1mva/NumOscillation ==
  Ground2 : powerlib/Elements/Ground  LConnTagsString=a
  "RLC " : powerlib/Elements/Parallel RLC Branch  LConnTagsString=a  RConnTagsString=__new0  BranchType=R  Resistance=10e6  Inductance=inf  SetiL0=off  InitialCurrent=0  Capacitance=10e-6  Setx0=off  InitialVoltage=0  Measurements=None
  RLC1 : powerlib/Elements/Parallel RLC Branch  LConnTagsString=a  RConnTagsString=__new0  BranchType=R  Resistance=10e6  Inductance=inf  SetiL0=off  InitialCurrent=0  Capacitance=10e-6  Setx0=off  InitialVoltage=0  Measurements=None
  RLC2 : powerlib/Elements/Parallel RLC Branch  LConnTagsString=a  RConnTagsString=__new0  BranchType=R  Resistance=10e6  Inductance=inf  SetiL0=off  InitialCurrent=0  Capacitance=10e-6  Setx0=off  InitialVoltage=0  Measurements=None
  RLC3 : powerlib/Elements/Parallel RLC Branch  LConnTagsString=a  RConnTagsString=__new0  BranchType=R  Resistance=10e-3  Inductance=inf  SetiL0=off  InitialCurrent=0  Capacitance=0  Setx0=off  InitialVoltage=0  Measurements=None
  RLC4 : powerlib/Elements/Parallel RLC Branch  LConnTagsString=a  RConnTagsString=__new0  BranchType=R  Resistance=10e-3  Inductance=inf  SetiL0=off  InitialCurrent=0  Capacitance=0  Setx0=off  InitialVoltage=0  Measurements=None
  RLC5 : powerlib/Elements/Parallel RLC Branch  LConnTagsString=a  RConnTagsString=__new0  BranchType=R  Resistance=10e-3  Inductance=inf  SetiL0=off  InitialCurrent=0  Capacitance=0  Setx0=off  InitialVoltage=0  Measurements=None
  A : PMIOPort  Port=1  Side=Left
  B : PMIOPort  Port=2  Side=Left
  C : PMIOPort  Port=3  Side=Left
  connections:
  "RLC "/RConn1 -- RLC1/RConn1 -- Ground2/LConn1 -- RLC2/RConn1
  "RLC "/LConn1 -- RLC5/RConn1
  RLC1/LConn1 -- RLC4/RConn1
  RLC3/RConn1 -- RLC2/LConn1
  A/RConn1 -- RLC3/LConn1
  B/RConn1 -- RLC4/LConn1
  C/RConn1 -- RLC5/LConn1

== system NGGenset_Test_System/SM_Master/Generator/GenSet_4MVA_copy1mva/Simulated Generator Controller 3.5 MW ==
  Pref : Inport
  Qref : Inport  Port=2
  mode : Inport  Port=3
  set_vtref : Inport  Port=4
  set_wref : Inport  Port=5
  gen_m : Inport  Port=6
  Bus Selector1 : BusSelector  OutputSignals="Output active power   Peo (pu),Output reactive power  Qeo (pu)"
  Multiport Switch : MultiPortSwitch
  Mux1 : Mux  Inputs=2
  Mux2 : Mux  Inputs=2
  Mux3 : Mux  Inputs=2
  PQ control : Subsystem
  PV control : Subsystem
  "wref, Vref" : Outport
  wires:
  Multiport Switch/1 -> "wref, Vref"/1
  mode/1 -> Multiport Switch/1
  Qref/1 -> PQ control/3(Q_ref (pu))
  set_wref/1 -> Mux3/1
  Bus Selector1/2 -> PQ control/4(Q (pu))  "<Output reactive power  Qeo (pu)>"
  Pref/1 -> PV control/1(P_ref (pu)), PQ control/1(P_ref (pu))
  Mux3/1 -> Multiport Switch/4
  Mux2/1 -> Multiport Switch/3
  Mux1/1 -> Multiport Switch/2
  set_vtref/1 -> Mux3/2, Mux2/2
  PV control/1(w_ref (pu)) -> Mux2/1
  PQ control/2(V_ref (pu)) -> Mux1/2
  PQ control/1(w_ref (pu)) -> Mux1/1
  gen_m/1 -> Bus Selector1/1
  Bus Selector1/1 -> PV control/2(P (pu)), PQ control/2(P (pu))  "<Output active power   Peo (pu)>"

== system NGGenset_Test_System/SM_Master/Generator/GenSet_4MVA_copy1mva/StabilityL ==
  Constant Load : powerlib/Elements/Three-Phase Parallel RLC Load  LConnTagsString=A|B|C  Configuration=Y (grounded)  NominalVoltage=v  NominalFrequency=60  ActivePower=kVA*1E3*pf  InductivePower=kVA*1E3*sqrt(1-pf^2)  CapacitivePower=0  Measurements=None  LoadType=constant Z
  A : PMIOPort  Port=1  Side=Left
  B : PMIOPort  Port=2  Side=Left
  C : PMIOPort  Port=3  Side=Left
  connections:
  C/RConn1 -- Constant Load/LConn3
  B/RConn1 -- Constant Load/LConn2
  A/RConn1 -- Constant Load/LConn1

== system NGGenset_Test_System/SM_Master/Generator/NG GenSet_3.5MVA_09212015/3.5MVA Generator with  Primary Controllers1 ==
  wref : Inport
  Vtref : Inport  Port=2
  Enable : Inport  Port=3
  w_meas_Woodward : Inport  Port=4
  V_meas_Woodward : Inport  Port=5
  Woodward_Enable : Inport  Port=6
  Bus Creator1 : BusCreator
  Bus Creator3 : BusCreator  Inputs=3
  Bus Selector : BusSelector  OutputSignals=Vf_before,Vf_after
  NG Engine Speed & Voltage Control fast : Subsystem
  Synchronous Machine pu Fundamental : powerlib/Machines/Synchronous Machine pu Fundamental  PresetModel=No  MechanicalLoad=Mechanical power Pm  ShowDetailedParameters=on  RotorType=Salient-pole  NominalParameters=[3.5e+006 13800 60]  Stator=[0.008979 0.05 2.35 1.72]  Field=[0.00206 0.511]  Dampers2=[0.0652, 0.5134, 0.0287, 0.2553, 7.765e-3, 0.9167 ]  Dampers1=[0.2826 3.738 0.02545 0.2392]  Mechanical=[0.3468 0.009238 2]  PolePairs=2  InitialConditions="[ -99  0  0  0  0  0  0  0  0 ]"  SetSaturation=off  Saturation=[0.6404,0.7127,0.8441,0.9214,0.9956,1.082,1.19,1.316,1.457;0.7,0.7698,0.8872,0.9466,0.9969,1.046,1.1,1.151,1.201]  Units=per unit fundamental parameters  LoadFlowParameters=[1,0,0,0,0]  TsPowergui=0  TsBlock=-1  IterativeModel=Forward Euler  BusType=swing  Pref=0  Qref=0  Qmin=-inf  Qmax=inf  PLF=0  QLF=0
  A : PMIOPort  Port=1  Side=Right
  B : PMIOPort  Port=2  Side=Right
  C : PMIOPort  Port=3  Side=Right
  m : Outport
  Primary : Outport  Port=2
  Thermal data : Outport  Port=3
  wires:
  Woodward_Enable/1 -> NG Engine Speed & Voltage Control fast/7(Woodward Enable)
  Bus Creator3/1 -> Bus Creator1/2  "Vf"
  Bus Selector/2 -> Bus Creator3/3  "<Vf_after>"
  Bus Selector/1 -> Bus Creator3/2  "<Vf_before>"
  NG Engine Speed & Voltage Control fast/5(Misc) -> Bus Selector/1
  Bus Creator1/1 -> Primary/1
  NG Engine Speed & Voltage Control fast/4(w) -> Bus Creator1/4  "w"
  NG Engine Speed & Voltage Control fast/3(Vt) -> Bus Creator1/3  "vt"
  V_meas_Woodward/1 -> NG Engine Speed & Voltage Control fast/6(V_meas_Wood)
  w_meas_Woodward/1 -> NG Engine Speed & Voltage Control fast/5(w_meas_Wood)
  Synchronous Machine pu Fundamental/1 -> m/1, NG Engine Speed & Voltage Control fast/4(m)
  Enable/1 -> NG Engine Speed & Voltage Control fast/3(Generator Enable)
  NG Engine Speed & Voltage Control fast/1(Pm) -> Synchronous Machine pu Fundamental/1, Bus Creator1/1  "Pm"
  NG Engine Speed & Voltage Control fast/2(Vf) -> Synchronous Machine pu Fundamental/2, Bus Creator3/1  "vf"
  wref/1 -> NG Engine Speed & Voltage Control fast/1(wref)
  Vtref/1 -> NG Engine Speed & Voltage Control fast/2(Vtref)
  NG Engine Speed & Voltage Control fast/6(Themal data) -> Thermal data/1
  connections:
  Synchronous Machine pu Fundamental/RConn1 -- A/RConn1
  Synchronous Machine pu Fundamental/RConn2 -- B/RConn1
  Synchronous Machine pu Fundamental/RConn3 -- C/RConn1

== system NGGenset_Test_System/SM_Master/Generator/NG GenSet_3.5MVA_09212015/Interface between Woodward Controller and simated generator ==
  note: Note: This may need a different scaling because it is the reference signal.
      | Reference has to be between 0.95 and 1.05 pu in order to be in tolerance.
  Woodward for wref : Inport
  Woodward for Vref : Inport  Port=2
  Add2 : Sum
  Add3 : Sum
  Gain2 : Gain
  Gain3 : Gain
  Mux1 : Mux  Inputs=2
  Vref_set : Constant  Value=0
  wref_set : Constant  Value=0
  wref,Vref : Outport
  wires:
  Gain2/1 -> Add2/1  "bias"
  Add2/1 -> Mux1/1
  wref_set/1 -> Add2/2
  Gain3/1 -> Add3/1  "bias"
  Vref_set/1 -> Add3/2
  Add3/1 -> Mux1/2
  Woodward for wref/1 -> Gain2/1
  Mux1/1 -> wref,Vref/1  "hardware"
  Woodward for Vref/1 -> Gain3/1

== system NGGenset_Test_System/SM_Master/Generator/NG GenSet_3.5MVA_09212015/Simulated Generator Controller 3.5 MW ==
  Pref : Inport
  Qref : Inport  Port=2
  mode : Inport  Port=3
  set_vtref : Inport  Port=4
  set_wref : Inport  Port=5
  gen_m : Inport  Port=6
  Bus Selector1 : BusSelector  OutputSignals="Output active power   Peo (pu),Output reactive power  Qeo (pu)"
  Multiport Switch1 : MultiPortSwitch  DiagnosticForDefault=Warning
  Mux1 : Mux  Inputs=2
  Mux2 : Mux  Inputs=2
  Mux3 : Mux  Inputs=2
  PQ control : Subsystem
  PV control : Subsystem
  "wref, Vref" : Outport
  wires:
  Bus Selector1/1 -> PQ control/2(P (pu)), PV control/2(P (pu))  "<Output active power   Peo (pu)>"
  gen_m/1 -> Bus Selector1/1
  PQ control/1(w_ref (pu)) -> Mux1/1
  PQ control/2(V_ref (pu)) -> Mux1/2
  PV control/1(w_ref (pu)) -> Mux2/1
  set_vtref/1 -> Mux2/2, Mux3/2
  Mux1/1 -> Multiport Switch1/2
  Mux2/1 -> Multiport Switch1/3
  Mux3/1 -> Multiport Switch1/4
  Bus Selector1/2 -> PQ control/4(Q (pu))  "<Output reactive power  Qeo (pu)>"
  mode/1 -> Multiport Switch1/1
  Multiport Switch1/1 -> "wref, Vref"/1
  Qref/1 -> PQ control/3(Q_ref (pu))
  Pref/1 -> PQ control/1(P_ref (pu)), PV control/1(P_ref (pu))
  set_wref/1 -> Mux3/1

== system NGGenset_Test_System/SM_Master/Generator/NG GenSet_3.5MVA_09212015/StabilityL ==
  Constant Load : powerlib/Elements/Three-Phase Parallel RLC Load  LConnTagsString=A|B|C  Configuration=Y (grounded)  NominalVoltage=v  NominalFrequency=60  ActivePower=kVA*1E3*pf  InductivePower=kVA*1E3*sqrt(1-pf^2)  CapacitivePower=0  Measurements=None  LoadType=constant Z
  A : PMIOPort  Port=1  Side=Left
  B : PMIOPort  Port=2  Side=Left
  C : PMIOPort  Port=3  Side=Left
  connections:
  A/RConn1 -- Constant Load/LConn1
  B/RConn1 -- Constant Load/LConn2
  C/RConn1 -- Constant Load/LConn3

== system NGGenset_Test_System/SM_Master/Generator/Woodward Inputs/Speed_System ==
  In1 : Inport
  Clock1 : Clock
      settings: DisableCoverage=on
  Duty : Constant  DisableCoverage=on  Value=0.5
  Gain1 : Gain  Gain=5
  Gain3 : Gain  Gain=5
  Gain4 : Gain  Gain=1800
  Output : Trigonometry
  Product1 : Product  DisableCoverage=on  SaturateOnIntegerOverflow=on  InputSameDT=on  OutDataTypeStr=Inherit: Same as first input
  Product3 : Product  DisableCoverage=on  SaturateOnIntegerOverflow=on  InputSameDT=on  OutDataTypeStr=Inherit: Same as first input
  RTE Conversion : rteventslib/Signal Attributes/RTE Conversion  inputdatatype=RTE Boolean  outputdatatype=Double  compensation=Disabled  nbMaxEvents=10  sampleTime=Ts
  RTE SPWM : rteventslib/Sources/RTE SPWM  NumberPhases=1-ph  CenterAlignmentMode=On  MaxFreq=inf  MinFreq=0  EnablingPort=off  ComplementaryMode=off  SpaceVector=off  RiseTimeDelay=0  MaxEvents=10  SampleTime=Ts
  initialFreq : Constant  DisableCoverage=on  Value=2*pi
  Out1 : Outport
  wires:
  Gain1/1 -> Out1/1
  RTE Conversion/1 -> Gain1/1
  Duty/1 -> RTE SPWM/2
  RTE SPWM/1 -> RTE Conversion/1
  In1/1 -> Gain4/1
  Output/1 -> Gain3/1
  Gain4/1 -> RTE SPWM/1, Product3/2
  Product3/1 -> Product1/2
  initialFreq/1 -> Product3/1
  Clock1/1 -> Product1/1
  Product1/1 -> Output/1

== system NGGenset_Test_System/SM_Master/Generator/Woodward Inputs/Speed_System1 ==
  In1 : Inport
  Clock1 : Clock
      settings: DisableCoverage=on
  Duty : Constant  DisableCoverage=on  Value=0.5
  Gain1 : Gain  Gain=5
  Gain3 : Gain  Gain=5
  Gain4 : Gain  Gain=1800
  Output : Trigonometry
  Product1 : Product  DisableCoverage=on  SaturateOnIntegerOverflow=on  InputSameDT=on  OutDataTypeStr=Inherit: Same as first input
  Product3 : Product  DisableCoverage=on  SaturateOnIntegerOverflow=on  InputSameDT=on  OutDataTypeStr=Inherit: Same as first input
  RTE Conversion : rteventslib/Signal Attributes/RTE Conversion  inputdatatype=RTE Boolean  outputdatatype=Double  compensation=Disabled  nbMaxEvents=10  sampleTime=Ts
  RTE SPWM : rteventslib/Sources/RTE SPWM  NumberPhases=1-ph  CenterAlignmentMode=On  MaxFreq=inf  MinFreq=0  EnablingPort=off  ComplementaryMode=off  SpaceVector=off  RiseTimeDelay=0  MaxEvents=10  SampleTime=Ts
  initialFreq : Constant  DisableCoverage=on  Value=2*pi
  Out1 : Outport
  wires:
  Gain1/1 -> Out1/1
  RTE Conversion/1 -> Gain1/1
  Duty/1 -> RTE SPWM/2
  RTE SPWM/1 -> RTE Conversion/1
  In1/1 -> Gain4/1
  Output/1 -> Gain3/1
  Gain4/1 -> RTE SPWM/1, Product3/2
  Product3/1 -> Product1/2
  initialFreq/1 -> Product3/1
  Clock1/1 -> Product1/1
  Product1/1 -> Output/1

== system NGGenset_Test_System/SM_Master/Generator/Woodward Outputs/DIO - Gr3 ==
  Dout : Inport
  Bus Creator : BusCreator  Inputs=2
  Bus Selector : BusSelector  OutputSignals=DI_CH00-07  OutputAsBus=on
  Bus Selector1 : BusSelector  OutputSignals=DI_CH08-15  OutputAsBus=on
  Conditioning : Subsystem
  Conditioning1 : Subsystem
  DigitalIn : rtio_opalrt_common/DigitalIn  CtrlName='OpCtrl'  portNb=5  FcnNos=Slot 3 Module A Subsection 1  size=1  maxcount=8  count=8  sampleTime=0  numchan=8
      settings: AttributesFormatString=%<CtrlName>
  DigitalIn1 : rtio_opalrt_common/DigitalIn  CtrlName='OpCtrl'  portNb=6  FcnNos=Slot 3 Module A Subsection 2  size=1  maxcount=8  count=8  sampleTime=0  numchan=8
      settings: AttributesFormatString=%<CtrlName>
  DigitalOut : rtio_opalrt_common/DigitalOut  CtrlName='OpCtrl'  portNb=5  FcnNos=Slot 3 Module B Subsection 1  size=1  maxcount=8  count=8  numchan=8
      settings: AttributesFormatString=%<CtrlName>
  DigitalOut1 : rtio_opalrt_common/DigitalOut  CtrlName='OpCtrl'  portNb=6  FcnNos=Slot 3 Module B Subsection 2  size=1  maxcount=8  count=8  numchan=8
      settings: AttributesFormatString=%<CtrlName>
  Terminator{1,3,5..6} (4 alike) : Terminator
  DIn : Outport
  wires:
  DigitalOut/1 -> Terminator3/1
  DigitalOut1/1 -> Terminator1/1
  Dout/1 -> Bus Selector/1, Bus Selector1/1
  Bus Selector/1 -> DigitalOut/1
  Bus Selector1/1 -> DigitalOut1/1
  DigitalIn/2 -> Terminator5/1
  DigitalIn1/2 -> Terminator6/1
  DigitalIn/1 -> Conditioning/1(In1)  "DI_CH00-07"
  DigitalIn1/1 -> Conditioning1/1(In1)  "DI_CH08-15"
  Bus Creator/1 -> DIn/1
  Conditioning/1(Out1) -> Bus Creator/1
  Conditioning1/1(Out1) -> Bus Creator/2

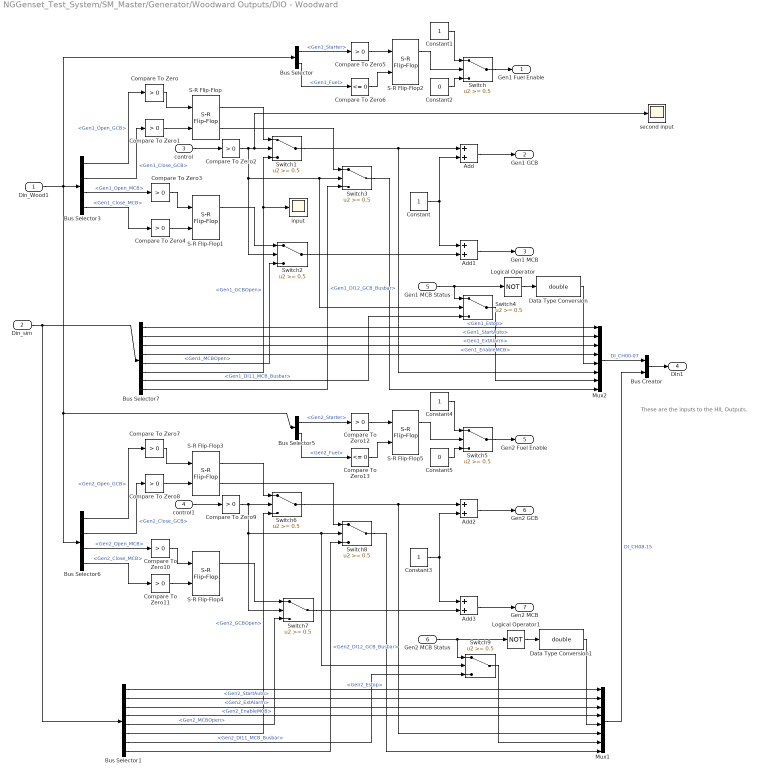
== system NGGenset_Test_System/SM_Master/Generator/Woodward Outputs/DIO - Woodward ==
  note: These are the inputs to
      | the HIL Outputs.
  Din_Wood1 : Inport
  Din_sim : Inport  Port=2
  control : Inport  Port=3
  control1 : Inport  Port=4
  Gen1 MCB Status : Inport  Port=5
  Gen2 MCB Status : Inport  Port=6
  Add{,1..3} (4 alike) : Sum
  Bus Creator : BusCreator  Inputs=2
  Bus Selector : BusSelector  OutputSignals=DI_CH00-07.Gen1_Starter,DI_CH00-07.Gen1_Fuel
  Bus Selector1 : BusSelector  OutputSignals=16 DOUT GR3.08-11.Gen2_Estop,16 DOUT GR3.08-11.Gen2_StartAuto,16 DOUT GR3.08-11.Gen2_ExtAlarm,16 DOUT GR3.08-11.Gen2_EnableMCB,16 DOUT GR3.12-15.Gen2_MCBOpen,16 DOUT GR3.12-15.Gen2_GCBOpen,16 DOUT GR3.12-15.Gen2_DI11_MCB_Busbar,16 DOUT GR3.12-15.Gen2_DI12_GCB_Busbar
  Bus Selector3 : BusSelector  OutputSignals=DI_CH00-07.Gen1_Open_GCB,DI_CH00-07.Gen1_Close_GCB,DI_CH00-07.Gen1_Open_MCB,DI_CH00-07.Gen1_Close_MCB
  Bus Selector5 : BusSelector  OutputSignals=DI_CH08-15.Gen2_Starter,DI_CH08-15.Gen2_Fuel
  Bus Selector6 : BusSelector  OutputSignals=DI_CH08-15.Gen2_Open_GCB,DI_CH08-15.Gen2_Close_GCB,DI_CH08-15.Gen2_Open_MCB,DI_CH08-15.Gen2_Close_MCB
  Bus Selector7 : BusSelector  OutputSignals=16 DOUT GR3.00-03.Gen1_Estop,16 DOUT GR3.00-03.Gen1_StartAuto,16 DOUT GR3.00-03.Gen1_ExtAlarm,16 DOUT GR3.00-03.Gen1_EnableMCB,16 DOUT GR3.04-07.Gen1_MCBOpen,16 DOUT GR3.04-07.Gen1_GCBOpen,16 DOUT GR3.04-07.Gen1_DI11_MCB_Busbar,16 DOUT GR3.04-07.Gen1_DI12_GCB_Busbar
  Compare To Zero{,1..5,7..12} (12 alike) : simulink/Logic and Bit Operations/Compare To Zero  relop=>  OutDataTypeStr=boolean
  Compare To Zero13 : simulink/Logic and Bit Operations/Compare To Zero  relop=<=  OutDataTypeStr=boolean
  Compare To Zero6 : simulink/Logic and Bit Operations/Compare To Zero  relop=<=  OutDataTypeStr=boolean
  Constant{,1,3..4} (4 alike) : Constant
  Constant2 : Constant  Value=0
  Constant5 : Constant  Value=0
  Data Type Conversion : DataTypeConversion  OutDataTypeStr=double
  Data Type Conversion1 : DataTypeConversion  OutDataTypeStr=double
  Logical Operator : Logic  Operator=NOT  AllPortsSameDT=off  OutDataTypeStr=boolean
  Logical Operator1 : Logic  Operator=NOT  AllPortsSameDT=off  OutDataTypeStr=boolean
  Mux1 : Mux  Inputs=8
  Mux2 : Mux  Inputs=8
  S-R Flip-Flop{,1,3..4} (4 alike) : simulink_extras/Flip Flops/S-R Flip-Flop  initial_condition=1
  S-R Flip-Flop2 : simulink_extras/Flip Flops/S-R Flip-Flop  initial_condition=0
  S-R Flip-Flop5 : simulink_extras/Flip Flops/S-R Flip-Flop  initial_condition=0
  Switch : Switch  Threshold=0.5
  Switch{1..4,6..9} (8 alike) : Switch  Threshold=0.5  OutDataTypeStr=double
      Switch8 settings: LockScale=on
  Switch5 : Switch  Threshold=0.5
  input : Scope
      settings: SaveName=ScopeData14
  "second input " : Scope
      settings: YMin=1  YMax=1  SaveName=ScopeData15
  Gen1 Fuel Enable : Outport
  Gen1 GCB : Outport  Port=2
  Gen1 MCB : Outport  Port=3
  DIn1 : Outport  Port=4
  Gen2 Fuel Enable : Outport  Port=5
  Gen2 GCB : Outport  Port=6
  Gen2 MCB : Outport  Port=7
  wires:
  Din_Wood1/1 -> Bus Selector3/1, Bus Selector/1, Bus Selector6/1, Bus Selector5/1
  control/1 -> Compare To Zero2/1
  Bus Creator/1 -> DIn1/1
  S-R Flip-Flop/1 -> Switch1/1
  Switch1/1 -> Add/1, Mux2/6
  Bus Selector3/1 -> Compare To Zero/1  "<Gen1_Open_GCB>"
  Compare To Zero/1 -> S-R Flip-Flop/1
  Compare To Zero1/1 -> S-R Flip-Flop/2
  Bus Selector3/4 -> Compare To Zero4/1  "<Gen1_Close_MCB>"
  Compare To Zero4/1 -> S-R Flip-Flop1/2
  Compare To Zero3/1 -> S-R Flip-Flop1/1
  S-R Flip-Flop1/1 -> Switch2/1
  Compare To Zero2/1 -> "second input "/1, Switch1/2, Switch2/2, Switch3/2, Switch4/2
  Switch2/1 -> Add1/2
  Mux1/1 -> Bus Creator/2  "DI_CH08-15"
  S-R Flip-Flop/2 -> Switch3/1
  Add/1 -> Gen1 GCB/1
  Add1/1 -> Gen1 MCB/1
  Constant/1 -> Add/2, Add1/1
  Bus Selector/1 -> Compare To Zero5/1  "<Gen1_Starter>"
  Bus Selector/2 -> Compare To Zero6/1  "<Gen1_Fuel>"
  S-R Flip-Flop2/1 -> Switch/2
  Compare To Zero5/1 -> S-R Flip-Flop2/1
  Constant2/1 -> Switch/3
  Constant1/1 -> Switch/1
  Compare To Zero6/1 -> S-R Flip-Flop2/2
  Switch/1 -> Gen1 Fuel Enable/1
  control1/1 -> Compare To Zero9/1
  S-R Flip-Flop3/1 -> Switch6/1
  Switch6/1 -> Add2/1, Mux1/6
  Bus Selector6/1 -> Compare To Zero7/1  "<Gen2_Open_GCB>"
  Compare To Zero7/1 -> S-R Flip-Flop3/1
  Compare To Zero8/1 -> S-R Flip-Flop3/2
  Bus Selector6/4 -> Compare To Zero11/1  "<Gen2_Close_MCB>"
  Compare To Zero11/1 -> S-R Flip-Flop4/2
  Bus Selector6/3 -> Compare To Zero10/1  "<Gen2_Open_MCB>"
  Compare To Zero10/1 -> S-R Flip-Flop4/1
  S-R Flip-Flop4/1 -> Switch7/1
  Bus Selector6/2 -> Compare To Zero8/1  "<Gen2_Close_GCB>"
  Compare To Zero9/1 -> Switch6/2, Switch7/2, Switch8/2, Switch9/2
  Switch7/1 -> Add3/2
  S-R Flip-Flop3/2 -> Switch8/1
  Add2/1 -> Gen2 GCB/1
  Add3/1 -> Gen2 MCB/1
  Constant3/1 -> Add2/2, Add3/1
  Bus Selector5/1 -> Compare To Zero12/1  "<Gen2_Starter>"
  Bus Selector5/2 -> Compare To Zero13/1  "<Gen2_Fuel>"
  S-R Flip-Flop5/1 -> Switch5/2
  Compare To Zero12/1 -> S-R Flip-Flop5/1
  Constant5/1 -> Switch5/3
  Constant4/1 -> Switch5/1
  Compare To Zero13/1 -> S-R Flip-Flop5/2
  Switch5/1 -> Gen2 Fuel Enable/1
  Bus Selector3/2 -> Compare To Zero1/1  "<Gen1_Close_GCB>"
  Bus Selector3/3 -> Compare To Zero3/1  "<Gen1_Open_MCB>"
  Bus Selector1/1 -> Mux1/1  "<Gen2_Estop>"
  Bus Selector1/2 -> Mux1/2  "<Gen2_StartAuto>"
  Bus Selector1/3 -> Mux1/3  "<Gen2_ExtAlarm>"
  Bus Selector1/4 -> Mux1/4  "<Gen2_EnableMCB>"
  Bus Selector1/5 -> Switch7/3  "<Gen2_MCBOpen>"
  Bus Selector1/6 -> Switch6/3  "<Gen2_GCBOpen>"
  Bus Selector7/1 -> Mux2/1  "<Gen1_Estop>"
  Bus Selector7/2 -> Mux2/2  "<Gen1_StartAuto>"
  Bus Selector7/3 -> Mux2/3  "<Gen1_ExtAlarm>"
  Bus Selector7/4 -> Mux2/4  "<Gen1_EnableMCB>"
  Bus Selector7/5 -> Switch2/3  "<Gen1_MCBOpen>"
  Bus Selector7/6 -> input/1, Switch1/3  "<Gen1_GCBOpen>"
  Mux2/1 -> Bus Creator/1  "DI_CH00-07"
  Din_sim/1 -> Bus Selector7/1, Bus Selector1/1
  Bus Selector7/7 -> Switch4/3  "<Gen1_DI11_MCB_Busbar>"
  Switch4/1 -> Mux2/7
  Bus Selector7/8 -> Switch3/3  "<Gen1_DI12_GCB_Busbar>"
  Switch3/1 -> Mux2/8
  Bus Selector1/7 -> Switch9/3  "<Gen2_DI11_MCB_Busbar>"
  Switch9/1 -> Mux1/7
  Bus Selector1/8 -> Switch8/3  "<Gen2_DI12_GCB_Busbar>"
  Switch8/1 -> Mux1/8
  Gen1 MCB Status/1 -> Logical Operator/1, Switch4/1
  Data Type Conversion/1 -> Mux2/5
  Logical Operator/1 -> Data Type Conversion/1
  Gen2 MCB Status/1 -> Logical Operator1/1, Switch9/1
  Logical Operator1/1 -> Data Type Conversion1/1
  Data Type Conversion1/1 -> Mux1/5

== system NGGenset_Test_System/SM_Master/Generator/Woodward Outputs/DOUT type config ==
  note: The Constants are used to select Digital Output type:
      | - 0: Time-Stamped Digital Output
      | - 1: Pulse-Width Modulated DIgital Output
  DataIn Send : rtio_opalrt_common/DataIn Send  CtrlName='OpCtrl'  FcnNos=11  width=1  portType=double  checkVersion=off  expectedId=0  expectedVersion=0  opComp=>=
      settings: AttributesFormatString=%<CtrlName>
  DataIn Send1 : rtio_opalrt_common/DataIn Send  CtrlName='OpCtrl'  FcnNos=12  width=1  portType=double  checkVersion=off  expectedId=0  expectedVersion=0  opComp=>=
      settings: AttributesFormatString=%<CtrlName>
  Subsection 3 DOUT type : Constant
  Subsection 4 DOUT type : Constant
  Terminator1 : Terminator
  Terminator2 : Terminator
  wires:
  Subsection 3 DOUT type/1 -> DataIn Send/1
  Subsection 4 DOUT type/1 -> DataIn Send1/1
  DataIn Send1/1 -> Terminator1/1
  DataIn Send/1 -> Terminator2/1

== system NGGenset_Test_System/SM_Master/Generator/Woodward Outputs/PWM IO - Gr3 ==
  PWMOut : Inport
  Bus Creator : BusCreator  Inputs=2
  Bus Creator1 : BusCreator  Inputs=2
  Bus Creator2 : BusCreator  Inputs=2
  Bus Selector : BusSelector  OutputSignals=FreqPWMOut16-23,DutyPWMOut16-23
  Bus Selector1 : BusSelector  OutputSignals=FreqPWMOut24-31,DutyPWMOut24-31
  Bus Selector2 : BusSelector  OutputSignals=16 PWMOUT GR3.Ch16-23,16 PWMOUT GR3.Ch24-31
  PWM In : rtio_opalrt_common/PWM In  CtrlName='OpCtrl'  portNb=9  FcnNos=Slot 3 Module A Subsection 3  maxCount=8  Count=8  sampleTime=0  numchan=8
      settings: AttributesFormatString=%<CtrlName>
  PWM In1 : rtio_opalrt_common/PWM In  CtrlName='OpCtrl'  portNb=10  FcnNos=Slot 3 Module A Subsection 4  maxCount=8  Count=8  sampleTime=0  numchan=8
      settings: AttributesFormatString=%<CtrlName>
  PWM Out : rtio_opalrt_common/PWM Out  CtrlName='OpCtrl'  portNb=9  FcnNos=Slot 3 Module B Subsection 3  size=64  maxcount=8  count=8  polarity=Active High  symMode=Symmetric  complementary=off  deadTime=0  numchan=8  loadnb=1  initphase=[0 0 0 0 0 0 0 0]
      settings: AttributesFormatString=%<CtrlName>
  PWM Out1 : rtio_opalrt_common/PWM Out  CtrlName='OpCtrl'  portNb=10  FcnNos=Slot 3 Module B Subsection 4  size=64  maxcount=8  count=8  polarity=Active High  symMode=Symmetric  complementary=off  deadTime=0  numchan=8  loadnb=2  initphase=[0 0 0 0 0 0 0 0]
      settings: AttributesFormatString=%<CtrlName>
  Terminator{,1,4..5} (4 alike) : Terminator
  PWMIn : Outport
  wires:
  Bus Selector/1 -> PWM Out/1  "<FreqPWMOut16-23>"
  Bus Selector/2 -> PWM Out/2  "<DutyPWMOut16-23>"
  PWM Out/1 -> Terminator/1
  Bus Selector1/1 -> PWM Out1/1  "<FreqPWMOut24-31>"
  Bus Selector1/2 -> PWM Out1/2  "<DutyPWMOut24-31>"
  PWM Out1/1 -> Terminator1/1
  PWMOut/1 -> Bus Selector2/1
  Bus Selector2/1 -> Bus Selector/1  "<Ch16-23>"
  Bus Creator/1 -> PWMIn/1
  Bus Creator1/1 -> Bus Creator/1  "PWMI_CH16-23"
  Bus Creator2/1 -> Bus Creator/2  "PWMI_CH24-31"
  PWM In1/3 -> Terminator5/1
  PWM In/3 -> Terminator4/1
  PWM In/1 -> Bus Creator1/1  "Freq"
  PWM In/2 -> Bus Creator1/2  "Duty"
  PWM In1/1 -> Bus Creator2/1  "Freq"
  PWM In1/2 -> Bus Creator2/2  "Duty"
  Bus Selector2/2 -> Bus Selector1/1  "<Ch24-31>"
